simulink model "filter_kalman"  (R2022b)
settings: Solver=FixedStepAuto  StartTime=0.0  StopTime=1000  RelTol=1e-3
settings Model: Creator=86134  LastModifiedBy=86134
settings SolverCC: ZeroCrossControl=DisableAll
settings DataIOCC: SaveOutput=off  SaveTime=off
settings GRTTargetCC: CombineOutputUpdateFcns=off  MatFileLogging=off

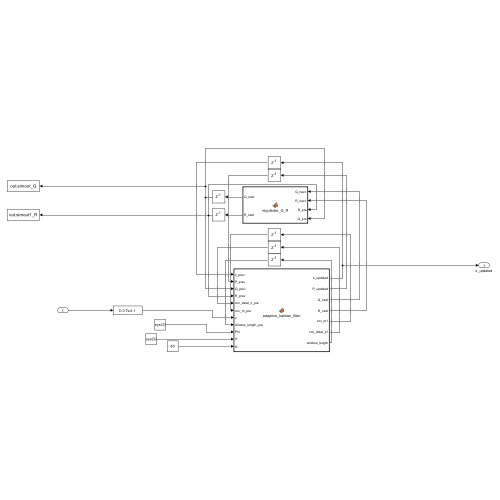
[thumbnail: Simulink's stored preview of the top-level diagram]
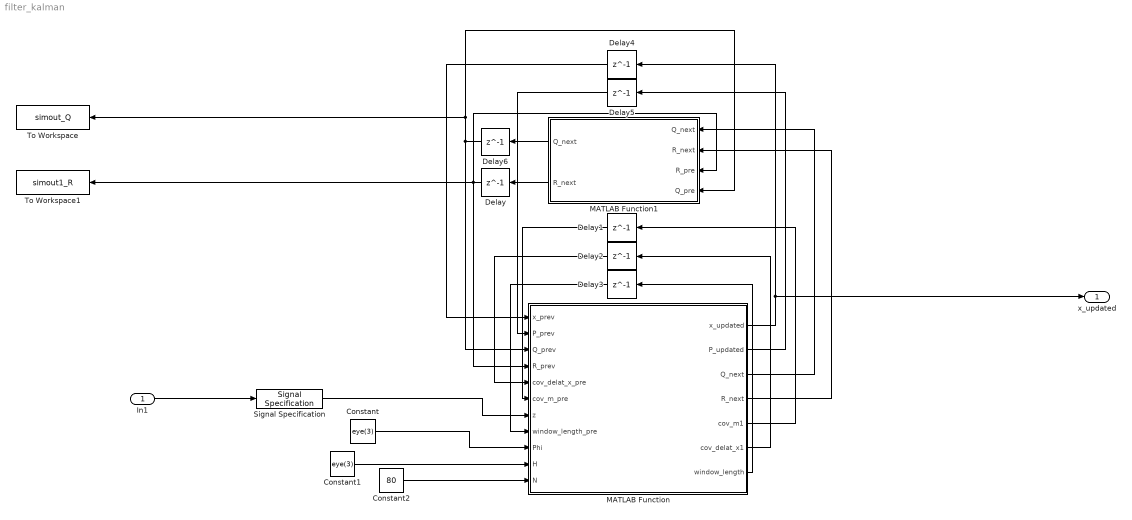
== system filter_kalman ==
  In1 : Inport
  Constant : Constant  Value=eye(3)
  Constant1 : Constant  Value=eye(3)
  Constant2 : Constant  Value=80
  Delay : Delay  DelayLength=1  InitialCondition=0.1*eye(3)
  Delay1 : Delay  DelayLength=1  InitialCondition=0.1.*eye(3)
  Delay2 : Delay  DelayLength=1  InitialCondition=0.1.*eye(3)
  Delay3 : Delay  DelayLength=1  InitialCondition=0
  Delay4 : Delay  DelayLength=1  InitialCondition="[101.325;  142.73;321.7924]"
  Delay5 : Delay  DelayLength=1  InitialCondition=0.1.*eye(3)
  Delay6 : Delay  DelayLength=1  InitialCondition=zeros(3)
  MATLAB Function : MATLAB Function  TreatAsAtomicUnit=on
  MATLAB Function1 : MATLAB Function  TreatAsAtomicUnit=on
  Signal Specification : SignalSpecification  Dimensions=3  SampleTime=0.1
  To Workspace : ToWorkspace  VariableName=simout_Q  SaveFormat=Timeseries  SampleTime=-1
  To Workspace1 : ToWorkspace  VariableName=simout1_R  SaveFormat=Timeseries  SampleTime=-1
  x_updated : Outport
  wires:
  In1/1 -> Signal Specification/1
  Signal Specification/1 -> MATLAB Function/7(z)
  MATLAB Function/1(x_updated) -> Delay4/1, x_updated/1
  MATLAB Function/2(P_updated) -> Delay5/1
  MATLAB Function/5(cov_m1) -> Delay1/1
  MATLAB Function/6(cov_delat_x1) -> Delay2/1
  MATLAB Function/7(window_length) -> Delay3/1
  Delay4/1 -> MATLAB Function/1(x_prev)
  Delay5/1 -> MATLAB Function/2(P_prev)
  Delay6/1 -> To Workspace/1, MATLAB Function1/4(Q_pre), MATLAB Function/3(Q_prev)
  Delay3/1 -> MATLAB Function/8(window_length_pre)
  Constant/1 -> MATLAB Function/9(Phi)
  Constant1/1 -> MATLAB Function/10(H)
  Constant2/1 -> MATLAB Function/11(N)
  Delay1/1 -> MATLAB Function/6(cov_m_pre)
  Delay2/1 -> MATLAB Function/5(cov_delat_x_pre)
  MATLAB Function1/1(Q_next) -> Delay6/1
  MATLAB Function1/2(R_next) -> Delay/1
  MATLAB Function/3(Q_next) -> MATLAB Function1/1("Q_next ")
  MATLAB Function/4(R_next) -> MATLAB Function1/2("R_next ")
  Delay/1 -> To Workspace1/1, MATLAB Function/4(R_prev), MATLAB Function1/3(R_pre)

== matlab function filter_kalman/MATLAB Function1 ==
  data: Q_next input; Q_next output; R_next input; R_pre input; Q_pre input; R_next output
function [Q_next,R_next] = regularize_Q_R(Q_next, R_next, R_pre,Q_pre)
    
   
    for i = 1:size(R_next, 1)
        if R_next(i, i) < 0
            R_next(i, i) = R_pre(i,i);
        end
    end
  
    for i = 1:size(Q_next, 1)
        if Q_next(i, i) < 0
            Q_next(i, i) = Q_pre(i,i);
        end
    end
%     R_next = 0.5 * (R_next + R_next'); % 强制对称
%     Q_next = 0.5 * (Q_next + Q_next');
    disp('Covariance Display:');
    disp([Q_next,R_next]);
    
end

== matlab function filter_kalman/MATLAB Function ==
  data: x_prev input; x_updated output; P_prev input; Q_prev input; R_prev input; cov_delat_x_pre input; cov_m_pre input; z input; window_length_pre input; Phi input; H input; N input; P_updated output; Q_next output; R_next output; cov_m1 output; cov_delat_x1 output; window_length output
function [x_updated, P_updated, Q_next, R_next, cov_m1, cov_delat_x1, window_length] = adaptive_kalman_filter(x_prev, P_prev, Q_prev, R_prev, cov_delat_x_pre, cov_m_pre, z, window_length_pre, Phi, H, N)
    persistent memory;
    if isempty(memory)
        memory.m_history = zeros(size(cov_m_pre, 1), N);  % 预分配固定大小的数组
        memory.delta_x_history = zeros(size(cov_delat_x_pre, 1), N);  % 预分配固定大小的数组
        memory.index = 0;  % 用于跟踪当前窗口的位置
    end

    % 预测
    x_predicted = Phi * x_prev;
    P_predicted = Phi * P_prev * Phi' + Q_prev;

    % 更新
    K = P_predicted * H' / (H * P_predicted * H' + R_prev);
    x_updated = x_predicted + K * (z - H * x_predicted);
    P_updated = (eye(size(P_predicted)) - K * H) * P_predicted;

    % 计算当前时间步的残差和状态校正
    m_k = z - H * x_predicted;
    delta_x_k = x_updated - x_predicted;

    % 更新窗口长度
    window_length = window_length_pre + 1;
    window_length = min(N, window_length);

    % 更新历史数据存储
    memory.index = memory.index + 1;
    if memory.index > N
        memory.index = 1;  
    end
    memory.m_history(:, memory.index) = m_k; 
    memory.delta_x_history(:, memory.index) = delta_x_k;


    %window_length=1;
    if window_length < N
        % 初始阶段：使用批量计算方法
        cov_m1 = cov_m_pre;
        cov_delat_x1 = cov_delat_x_pre;
        R_next = R_prev;
        Q_next = Q_prev;
    elseif window_length_pre == N - 1  % 标志着第一次数据点数达到了窗口长度
        cov_m1 = (1 / window_length) * (memory.m_history * memory.m_history');
        cov_delat_x1 = (1 / window_length) * (memory.delta_x_history * memory.delta_x_history');
        R_next = cov_m1 - H * P_predicted * H';
        Q_next = cov_delat_x1 + P_updated - Phi * P_prev * Phi';
    else
        % 稳定阶段：使用递归更新方法
        cov_m1 = N / (N + 1) * cov_m_pre + 1 / (N + 1) * (m_k * m_k');
        cov_delat_x1 = N / (N + 1) * cov_delat_x_pre + 1 / (N + 1) * (delta_x_k * delta_x_k');
        R_next = cov_m1 - H * P_predicted * H';
        Q_next = cov_delat_x1 + P_updated - Phi * P_prev * Phi';
    end
